simulink model "model_nivel_0"  (R2023a)
settings: Solver=VariableStepAuto  StartTime=0.0  StopTime=15.0  RelTol=1e-3
InitFcn:
  | parametros;
values from neighbouring files (symbols this model uses):
  T_s0 = 0.001    [parametros.m]
undefined symbols (not defined in the file or in its folder): parametros
settings Model: PacingRate=0.560000  Creator=Usuario  LastModifiedBy=Usuario

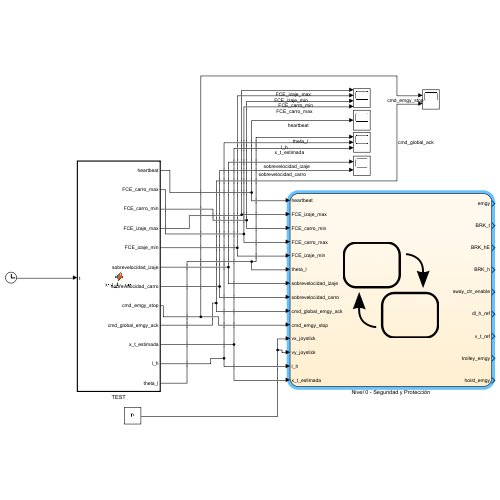
[thumbnail: Simulink's stored preview of the top-level diagram]
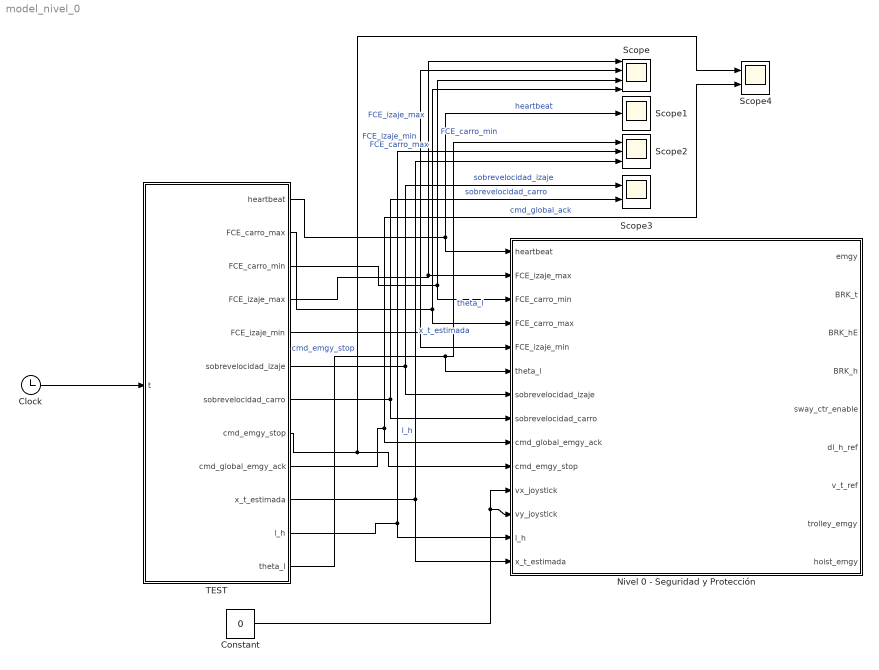
== system model_nivel_0 ==
  Clock : Clock
  Constant : Constant  Value=0
  Nivel 0 - Seguridad y Protección : Stateflow chart  InitFcn=parametros;  TreatAsAtomicUnit=on  SystemSampleTime=T_s0
  Scope : Scope  NumInputPorts=4
  Scope1 : Scope
  Scope2 : Scope  NumInputPorts=3
  Scope3 : Scope  NumInputPorts=2
  Scope4 : Scope  NumInputPorts=2
  TEST : MATLAB Function  TreatAsAtomicUnit=on
  wires:
  TEST/1(heartbeat) -> Scope1/1, Nivel 0 - Seguridad y Protección/1(heartbeat)  "heartbeat"
  Clock/1 -> TEST/1(t)
  TEST/2(FCE_carro_max) -> Scope/4, Nivel 0 - Seguridad y Protección/4(FCE_carro_max)  "FCE_carro_max"
  TEST/3(FCE_carro_min) -> Scope/3, Nivel 0 - Seguridad y Protección/3(FCE_carro_min)  "FCE_carro_min"
  TEST/4(FCE_izaje_max) -> Scope/1, Nivel 0 - Seguridad y Protección/2(FCE_izaje_max)  "FCE_izaje_max"
  TEST/6(sobrevelocidad_izaje) -> Nivel 0 - Seguridad y Protección/7(sobrevelocidad_izaje), Scope3/1  "sobrevelocidad_izaje"
  TEST/12(theta_l) -> Scope2/1, Nivel 0 - Seguridad y Protección/6(theta_l)  "theta_l"
  TEST/7(sobrevelocidad_carro) -> Nivel 0 - Seguridad y Protección/8(sobrevelocidad_carro), Scope3/2  "sobrevelocidad_carro"
  TEST/8(cmd_emgy_stop) -> Nivel 0 - Seguridad y Protección/10(cmd_emgy_stop), Scope4/1  "cmd_emgy_stop"
  TEST/9(cmd_global_emgy_ack) -> Nivel 0 - Seguridad y Protección/9(cmd_global_emgy_ack), Scope4/2  "cmd_global_ack"
  TEST/10(x_t_estimada) -> Nivel 0 - Seguridad y Protección/14(x_t_estimada), Scope2/3  "x_t_estimada"
  TEST/11(l_h) -> Nivel 0 - Seguridad y Protección/13(l_h), Scope2/2  "l_h"
  Constant/1 -> Nivel 0 - Seguridad y Protección/11(vx_joystick), Nivel 0 - Seguridad y Protección/12(vy_joystick)
  TEST/5(FCE_izaje_min) -> Scope/2, Nivel 0 - Seguridad y Protección/5(FCE_izaje_min)  "FCE_izaje_min"

== matlab function model_nivel_0/TEST ==
  data: t input; heartbeat output; FCE_carro_max output; FCE_carro_min output; FCE_izaje_max output; FCE_izaje_min output; sobrevelocidad_izaje output; sobrevelocidad_carro output; cmd_emgy_stop output; cmd_global_emgy_ack output; x_t_estimada output; l_h output; theta_l output
function [heartbeat, FCE_carro_max, FCE_carro_min, FCE_izaje_max, FCE_izaje_min, ...
          sobrevelocidad_izaje, sobrevelocidad_carro, cmd_emgy_stop, cmd_global_emgy_ack, ...
          x_t_estimada, l_h, theta_l] = test_loader(t)

% ============================================================
%  SELECCION DE TEST - habilitar solo uno
% ============================================================
TEST_normal          = true;
TEST_heartbeat_fail  = false; % OK
TEST_emgy_carro_max  = false; % OK
TEST_emgy_carro_min  = false; % OK
TEST_emgy_izaje_max  = false; % OK
TEST_emgy_izaje_min  = false; % OK
TEST_sobrevel_izaje  = false; % OK
TEST_sobrevel_carro  = false; % OK
TEST_emgy_stop       = true;

% ============================================================
%  VALORES BASE
% ============================================================
heartbeat            = logical(mod(floor(t / 0.2), 2));
FCE_carro_max        = false;
FCE_carro_min        = false;
FCE_izaje_max        = false;
FCE_izaje_min        = false;
sobrevelocidad_izaje = false;
sobrevelocidad_carro = false;
cmd_emgy_stop        = false;
cmd_global_emgy_ack  = false;
x_t_estimada         = 0.0;
l_h                  = 0.0;
theta_l              = 0.0;

% ============================================================
%  TEST_heartbeat_fail
% ============================================================
if TEST_heartbeat_fail
    if t > 5.0
        heartbeat = false;
    end
end

% ============================================================
%  TEST_emgy_carro_max
% ============================================================
if TEST_emgy_carro_max
    if t >= 2.0 && t < 10.0
        x_t_estimada  = 50.0;
        FCE_carro_max = true;
    elseif t >= 10.0
        x_t_estimada  = 40.0;
        FCE_carro_max = false;
    end
end

% ============================================================
%  TEST_emgy_carro_min
% ============================================================
if TEST_emgy_carro_min
    if t >= 2.0 && t < 10.0
        x_t_estimada  = -30.0;
        FCE_carro_min = true;
    elseif t >= 10.0
        x_t_estimada  = -20.0;
        FCE_carro_min = false;
    end
end

% ============================================================
%  TEST_emgy_izaje_max
% ============================================================
if TEST_emgy_izaje_max
    if t >= 2.0 && t < 10.0
        l_h           = 65.0;
        FCE_izaje_max = true;
    elseif t >= 10.0
        l_h           = 55.0;
        FCE_izaje_max = false;
    end
end

% ============================================================
%  TEST_emgy_izaje_min
% ============================================================
if TEST_emgy_izaje_min
    if t >= 2.0 && t < 10.0
        l_h           = 5.0;
        FCE_izaje_min = true;
    elseif t >= 10.0
        l_h           = 10.0;
        FCE_izaje_min = false;
    end
end

% ============================================================
%  TEST_sobrevel_izaje
% ============================================================
if TEST_sobrevel_izaje
    if (t >= 2.0 && t < 3.0) || (t >= 18.0 && t < 19.0)
        sobrevelocidad_izaje = true;
    end
end

% ============================================================
%  TEST_sobrevel_carro
% ============================================================
if TEST_sobrevel_carro
    if t >= 2.0 && t < 3.0
        sobrevelocidad_carro = true;
    end
end

% ============================================================
%  TEST_emgy_stop
% ============================================================
if TEST_emgy_stop
    if t >= 4.0 && t < 5.0
        cmd_emgy_stop = true;
    end
    if t >= 10.0
        cmd_global_emgy_ack = true;
    end
end

end

== stateflow chart model_nivel_0/Nivel 0 - Seguridad y Protección ==
  state Safety_Security_Control
    entry:
    emgy = false;
    watchdog_fail = false;
    heartbeat_prev = false;
    hoist_solved = false;
    trolley_solved = false;
    state Emergencies [parallel]
      settings: executionOrder=1
      state Stand_By
        entry:
        BRK_hE = true;
        BRK_h = true;
        BRK_t = true;
        hoist_solved = false;
        trolley_solved = false;
      state Trolley_Emgy
        entry:
        trolley_emgy = true;
        BRK_t = false;
        trolley_solved = false;
        v_t_ref = 0;
        state Init
        state Emgy_Switch_Min
          entry:
          BRK_t = true;
          during:
          v_t_ref = max([min([vx_joystick, 0.5]), 0]);
          dl_h_ref = vy_joystick;
        state Emgy_Switch_Max
          entry:
          BRK_t = true;
          during:
          v_t_ref = min([max([vx_joystick, -0.5]), 0]);
          dl_h_ref = vy_joystick;
        state Overspeed_Delay
        state Overspeed
          entry:
          sway_ctr_enable = false;
          state Init
          state Sway_Control
            entry:
            BRK_t = true;
            sway_ctr_enable = true;
          (default) -> Safety_Security_Control.Emergencies.Trolley_Emgy.Overspeed.Init
          Safety_Security_Control.Emergencies.Trolley_Emgy.Overspeed.Init -> Sway_Control : [after(3000, msec)]
        state Solved
          entry:
          trolley_emgy = false;
          trolley_solved = true;
        (default) -> Safety_Security_Control.Emergencies.Trolley_Emgy.Init
        Safety_Security_Control.Emergencies.Trolley_Emgy.Init -> Safety_Security_Control.Emergencies.Trolley_Emgy.Emgy_Switch_Min [order 1] : [FCE_carro_min && after(3000, msec)]
        Safety_Security_Control.Emergencies.Trolley_Emgy.Init -> Safety_Security_Control.Emergencies.Trolley_Emgy.Overspeed_Delay [order 3] : [sobrevelocidad_carro]
        Safety_Security_Control.Emergencies.Trolley_Emgy.Init -> Safety_Security_Control.Emergencies.Trolley_Emgy.Emgy_Switch_Max [order 2] : [FCE_carro_max && after(3000, msec)]
        Safety_Security_Control.Emergencies.Trolley_Emgy.Overspeed_Delay -> Safety_Security_Control.Emergencies.Trolley_Emgy.Overspeed : [after(3000, msec)]
        Safety_Security_Control.Emergencies.Trolley_Emgy.Emgy_Switch_Max -> Safety_Security_Control.Emergencies.Trolley_Emgy.Solved : [x_t_estimada <= x_t_safety_max]
        Safety_Security_Control.Emergencies.Trolley_Emgy.Emgy_Switch_Min -> Safety_Security_Control.Emergencies.Trolley_Emgy.Solved : [x_t_estimada >= x_t_safety_min]
        Safety_Security_Control.Emergencies.Trolley_Emgy.Overspeed -> Safety_Security_Control.Emergencies.Trolley_Emgy.Solved : [abs(theta_l*180/pi) <= 1]
      state Hoist_Emgy
        entry:
        hoist_emgy = true;
        BRK_hE = false;
        BRK_h = false;
        hoist_solved = false;
        dl_h_ref = 0;
        state Init
        state Emgy_Switch_Min
          entry:
          BRK_h = true;
          BRK_hE = true;
          during:
          v_t_ref = vx_joystick;
          dl_h_ref = max([min([vy_joystick, 0.5]), 0]);
        state Emgy_Switch_Max
          entry:
          BRK_h = true;
          BRK_hE = true;
          during:
          v_t_ref = vx_joystick;
          dl_h_ref = min([max([vy_joystick, -0.5]), 0]);
        state Overspeed_Delay
        state Overspeed
          entry:
          BRK_h = true;
          BRK_hE = true;
        state Solved
          entry:
          hoist_emgy = false;
          hoist_solved = true;
        (default) -> Safety_Security_Control.Emergencies.Hoist_Emgy.Init
        Safety_Security_Control.Emergencies.Hoist_Emgy.Init -> Safety_Security_Control.Emergencies.Hoist_Emgy.Emgy_Switch_Min [order 1] : [FCE_izaje_min && after(3000, msec)]
        Safety_Security_Control.Emergencies.Hoist_Emgy.Init -> Safety_Security_Control.Emergencies.Hoist_Emgy.Overspeed_Delay [order 3] : [sobrevelocidad_izaje]
        Safety_Security_Control.Emergencies.Hoist_Emgy.Init -> Safety_Security_Control.Emergencies.Hoist_Emgy.Emgy_Switch_Max [order 2] : [FCE_izaje_max && after(3000, msec)]
        Safety_Security_Control.Emergencies.Hoist_Emgy.Overspeed_Delay -> Safety_Security_Control.Emergencies.Hoist_Emgy.Overspeed : [after(3000, msec)]
        Safety_Security_Control.Emergencies.Hoist_Emgy.Emgy_Switch_Min -> Safety_Security_Control.Emergencies.Hoist_Emgy.Solved : [l_h >= l_h_safety_min]
        Safety_Security_Control.Emergencies.Hoist_Emgy.Emgy_Switch_Max -> Safety_Security_Control.Emergencies.Hoist_Emgy.Solved : [l_h <= l_h_safety_max]
        Safety_Security_Control.Emergencies.Hoist_Emgy.Overspeed -> Safety_Security_Control.Emergencies.Hoist_Emgy.Solved : [after(500, msec)]
      state Waiting_Global_Emgy_Ack
      state Global_Emgy
        entry:
        BRK_hE = false;
        BRK_t = false;
        BRK_h = false;
        emgy = true;
        during:
        v_t_ref = 0;
        dl_h_ref = 0;
      (default) -> Stand_By
      Stand_By -> Trolley_Emgy [order 3] : [FCE_carro_max || FCE_carro_min || sobrevelocidad_carro]
      Stand_By -> Global_Emgy [order 1] : [cmd_emgy_stop || watchdog_fail]
      Waiting_Global_Emgy_Ack -> Stand_By : [cmd_global_emgy_ack]{emgy=false;}
      Trolley_Emgy -> Stand_By : [trolley_solved]
      Stand_By -> Hoist_Emgy [order 2] : [FCE_izaje_min || FCE_izaje_max || sobrevelocidad_izaje]
      Hoist_Emgy -> Stand_By : [hoist_solved]
      Global_Emgy -> Waiting_Global_Emgy_Ack : [after(3000,msec)]
    state Watchdog [parallel]
      entry:
      counter = 0;
      heartbeat_prev = true;
      settings: executionOrder=2
      state Increase_counter
        entry:
        counter = counter + 1;
      state Init
      state Watchdog_Emgy
        entry:
        watchdog_fail = true;
      state Reset_Counter
        entry:
        counter = 0;
        heartbeat_prev = heartbeat;
      (default) -> Safety_Security_Control.Watchdog.Init
      Increase_counter -> Safety_Security_Control.Watchdog.Init
      Safety_Security_Control.Watchdog.Init -> Watchdog_Emgy [order 2] : [counter >= 5]
      Safety_Security_Control.Watchdog.Init -> Increase_counter [order 3] : [after(200, msec)]
      Safety_Security_Control.Watchdog.Init -> Reset_Counter [order 1] : [heartbeat_prev ~= heartbeat]
      Reset_Counter -> Safety_Security_Control.Watchdog.Init
  (default) -> Safety_Security_Control
  data: heartbeat input boolean; watchdog_fail local boolean size=1; counter local int8; heartbeat_prev local boolean; FCE_izaje_max input; FCE_carro_min input; FCE_carro_max input; FCE_izaje_min input; theta_l input; sobrevelocidad_izaje input; sobrevelocidad_carro input; emgy output; BRK_t output; BRK_hE output; BRK_h output; hoist_solved local; sway_ctr_enable output; dl_h_ref output; v_t_ref output; trolley_solved local; cmd_global_emgy_ack input; cmd_emgy_stop input; l_h_safety_min constant double =l_h_safety_min; vx_joystick input; vy_joystick input; x_t_safety_max constant double =x_t_safety_max; l_h input; l_h_safety_max constant double =l_h_safety_max; x_t_safety_min constant double =x_t_safety_min; x_t_estimada input; trolley_emgy output; hoist_emgy output
